simulink model "Project4_Simulink_individual"  (R2024b)
settings: Solver=ode4  StartTime=0.0  StopTime=3600  FixedStep=0.005  RelTol=1e-3
values from neighbouring files (symbols this model uses):
  ad = 2.5    [project4_code_final.m]
  b_capacity = 1500    [project4_code_final.m]
  c0 = 0.0041    [project4_code_final.m]
  c1 = 0.000066    (= 6.6e-05)    [project4_code_final.m]
  c_lambda = 50    [project4_code_final.m]
  calpha_front = 40000    [project4_code_final.m]
  calpha_rear = 40000    [project4_code_final.m]
  cd = 0.35    [project4_code_final.m]
  corner_factor = .95    (= 0.95)    [project4_code_final.m]
  eta_motor = 0.9    [project4_code_final.m]
  fyfrontmax = calpha_front * deg2rad(1)    [project4_code_final.m]
  fyrearmax = calpha_rear * deg2rad(1)    [project4_code_final.m]
  gratio = 2.5    [project4_code_final.m]
  i_gear_i = 0.005    [project4_code_final.m]
  inertia = 2000    [project4_code_final.m]
  ipt = 0.010    (= 0.01)    [project4_code_final.m]
  iw = 0.5 * 0.001* rw^2    (= 4.5e-05)    [project4_code_final.m]
  kd = 10000000    [project4_code_final.m]
  ki = 100    [project4_code_final.m]
  kp = 50000000    [project4_code_final.m]
  lambda_max = 0.1    [project4_code_final.m]
  lf = 1.0    (= 1)    [project4_code_final.m]
  lookahead_dist = 50    [project4_code_final.m]
  lookahead_dist_long = 100    [project4_code_final.m]
  lr = 1.5    [project4_code_final.m]
  mass = 1500    [project4_code_final.m]
  maxAlpha = 4 / 180 * pi    (= 0.0698131700798)    [project4_code_final.m]
  motor_torque_curve = [motor_rpm', motor_torque']    [project4_code_final.m]
  numSeries = 96    [project4_code_final.m]
  o_gear_i = 0.007    [project4_code_final.m]
  OCV = [0, 3.1,3.55,3.68,3.74,3.76,3.78,3.85,3.9,3.95,4.08,4.15]    [project4_code_final.m]
  omega0 = 0    [project4_code_final.m]
  psi0 = 0    [project4_code_final.m]
  r_internal = 0.1695    [project4_code_final.m]
  rho = 1.225    [project4_code_final.m]
  rw = 0.3    [project4_code_final.m]
  slope_angle_rad = atan(slope)    [project4_code_final.m]
  SOC = [0, 0.01,   .1,  .2,  .3,  .4,  .5,  .6, .7,  .8,  .9,   1]    [project4_code_final.m]
  soc_min = 0.1    [project4_code_final.m]
  T_lookahead = 0.3    [project4_code_final.m]
  tau_brakes = 50000    [project4_code_final.m]
  tire_mu = 1.0    (= 1)    [project4_code_final.m]
  v_batt = 350    [project4_code_final.m]
  vm = 1600    [project4_code_final.m]
  vx_threshold1 = 0.1    [project4_code_final.m]
  vxd = (max_motor_radps / gratio) * rw    [project4_code_final.m]
  vy0 = 0    [project4_code_final.m]
  wheelbase = lf + lr    (= 2.5)    [project4_code_final.m]
  x0 = 0    [project4_code_final.m]
  xpath = zeros(npts,1)    [project4_code_final.m]
  y0 = 0    [project4_code_final.m]
  ypath = zeros(npts,1)    [project4_code_final.m]
settings Model: Creator=btagl  LastModifiedBy=btagl

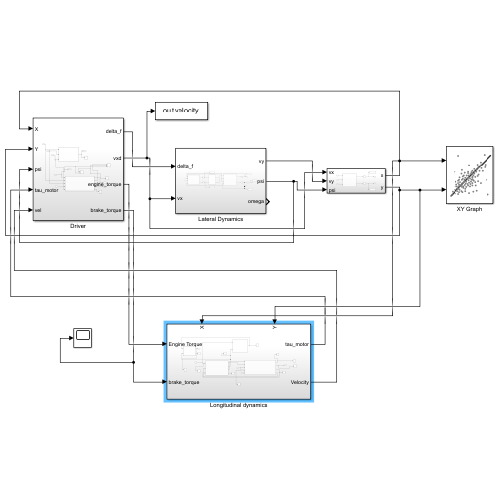
[thumbnail: Simulink's stored preview of the top-level diagram]
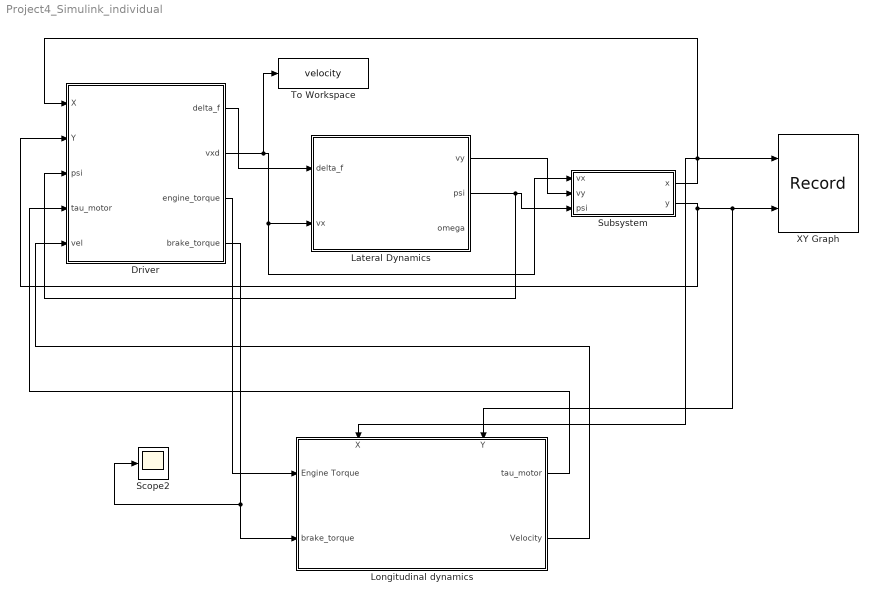
== system Project4_Simulink_individual ==
  Driver : Subsystem
  Lateral Dynamics : Subsystem
  Longitudinal dynamics : Subsystem
      settings: PortSchema="{\"entries\":[{\"content\":{\"sides\":[{\"content\":{\"connectorIds\":[\"In1\",\"In2\"]},\"type\":\"ConnectorPlacement.EquallySpacedRectSide\",\"uuid\":\"5c122f32-35de-43a9-a1a6-3743865a1a6c\"},{\"content\":{\"connectorIds\":[\"Out1\",\"Out2\"],\"side\":\"RIGHT\"},\"type\":\"ConnectorPlacement.EquallySpacedRectSide\",\"uuid\":\"4d44fb3e-15d5-4aaf-9487-b8861bfa0dad\"},{\"content\":{\"connectorIds\":[\"In3\",\"In4\"],\"side\":\"TOP\"},\"type\":\"ConnectorPlacement.EquallySpacedRectSide\",\"uuid\":\"e04a63df-9e81-4984-8ed3-9eee29f9a203\"}]},\"type\":\"ConnectorPlacement.EquallySpacedConnector\",\"uuid\":\"0a9d5385-60cd-4d4e-a9b3-28f03bd6bd4c\"}],\"packageUris\":[\"http://schema.mathworks.com/mf0/Connector/R2020b\"],\"version\":\"1.0\"}"
  Scope2 : Scope
  Subsystem : Subsystem
  To Workspace : ToWorkspace  VariableName=velocity  SaveFormat=Timeseries  SampleTime=-1
  XY Graph : Record  FileSettingsInternal="{\"entries\":[{\"content\":{\"excelSettings\":{\"content\":{},\"type\":\"Streamout.ExcelSettings\"}},\"type\":\"Streamout.FileSettingStorage\",\"uuid\":\"\"}],\"packageUris\":[\"http:\\/\\/schema.mathworks.com\\/mf0\\/streamout_blocks\\/R2020a\"],\"version\":\"1.0\"}"  Layout=[1 1]  SignalsInternal="{\"entries\":[{\"content\":{\"signals\":[{\"content\":{\"blockPath\":[],\"dimensions\":[1],\"domain\":\"\",\"lineColor\":\"#a2142f\",\"plots\":[ 1 ],\"port\":1,\"sid\":[\"\"],\"signalID\":1,\"signalName\":\"Subsystem:1\"},\"type\":\"RecordBlkView.Signal\",\"uuid\":\"\"},{\"content\":{\"blockPath\":[],\"dimensions\":[1],\"domain\":\"\",\"lineColor\":\"#139fff\",\"plots\":[ 1 ],\"port\":2,\"sid\":[\"\"],\"signalID\":2,\"signalName\":\"Subsystem:2\"},\"type\":\"RecordBlkView.Signal\",\"uuid\":\"\"}]},\"type\":\"RecordBlkView.InputSignals\",\"uuid\":\"\"}],\"packageUris\":[\"http:\\/\\/schema.mathworks.com\\/mf0\\/streamout_blocks\\/R2020a\"],\"version\":\"1.0\"}"  VisualizationBindings="{\"xyplotplugin\":{\"info\":[{\"series\":[{\"bindingParametersList\":[{\"parameter\":\"X-Axis\",\"signalID\":1,\"signalName\":\"Subsystem:1\"},{\"parameter\":\"Y-Axis\",\"signalID\":2,\"signalName\":\"Subsystem:2\"}],\"seriesID\":0}],\"subplotID\":1}]}}"  CompatibilityTag=XY
  wires:
  Subsystem/2(y) -> Driver/2(Y), XY Graph/2, Longitudinal dynamics/4(Y)
  Lateral Dynamics/2(psi) -> Driver/3(psi), Subsystem/3(psi)
  Lateral Dynamics/1(vy) -> Subsystem/2(vy)
  Driver/1(delta_f) -> Lateral Dynamics/1(delta_f)
  Driver/3(engine_torque) -> Longitudinal dynamics/1(Engine Torque)
  Driver/4(brake_torque) -> Scope2/1, Longitudinal dynamics/2(brake_torque)
  Longitudinal dynamics/1(tau_motor) -> Driver/4(tau_motor)
  Longitudinal dynamics/2(Velocity) -> Driver/5(vel)
  Driver/2(vxd) -> To Workspace/1, Subsystem/1(vx), Lateral Dynamics/2(vx)
  Subsystem/1(x) -> XY Graph/1, Longitudinal dynamics/3(X), Driver/1(X)

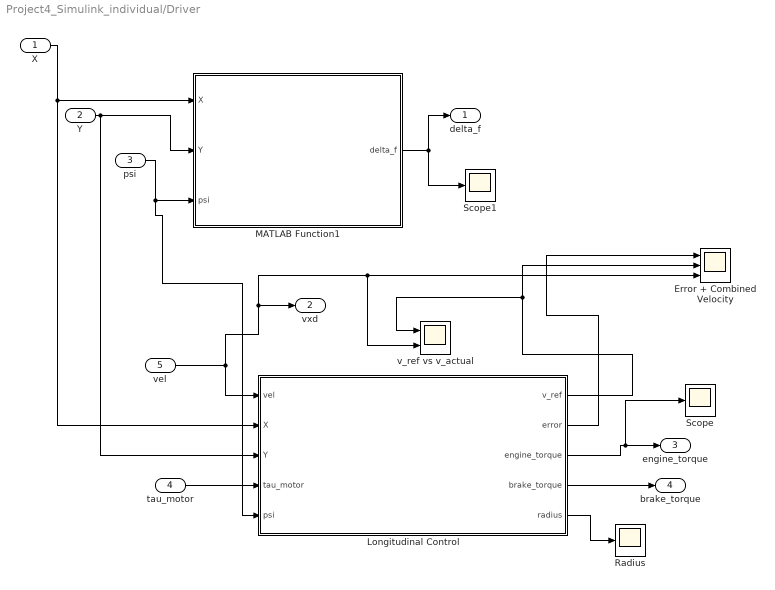
== system Project4_Simulink_individual/Driver ==
  X : Inport
  Y : Inport  Port=2
  psi : Inport  Port=3
  tau_motor : Inport  Port=4
  vel : Inport  Port=5
  Error + Combined Velocity : Scope  NumInputPorts=3
  Longitudinal Control : MATLAB Function  TreatAsAtomicUnit=on
  MATLAB Function1 : MATLAB Function  TreatAsAtomicUnit=on
  Radius : Scope
  Scope : Scope
  Scope1 : Scope
  v_ref vs v_actual : Scope  NumInputPorts=2
  delta_f : Outport
  vxd : Outport  Port=2
  engine_torque : Outport  Port=3
  brake_torque : Outport  Port=4
  wires:
  Y/1 -> Longitudinal Control/3(Y), MATLAB Function1/2(Y)
  X/1 -> Longitudinal Control/2(X), MATLAB Function1/1(X)
  MATLAB Function1/1(delta_f) -> delta_f/1, Scope1/1
  psi/1 -> Longitudinal Control/5(psi), MATLAB Function1/3(psi)
  tau_motor/1 -> Longitudinal Control/4(tau_motor)
  vel/1 -> Longitudinal Control/1(vel), vxd/1, v_ref vs v_actual/2, Error + Combined Velocity/3
  Longitudinal Control/1(v_ref) -> v_ref vs v_actual/1, Error + Combined Velocity/2
  Longitudinal Control/4(brake_torque) -> brake_torque/1
  Longitudinal Control/3(engine_torque) -> Scope/1, engine_torque/1
  Longitudinal Control/5(radius) -> Radius/1
  Longitudinal Control/2(error) -> Error + Combined Velocity/1

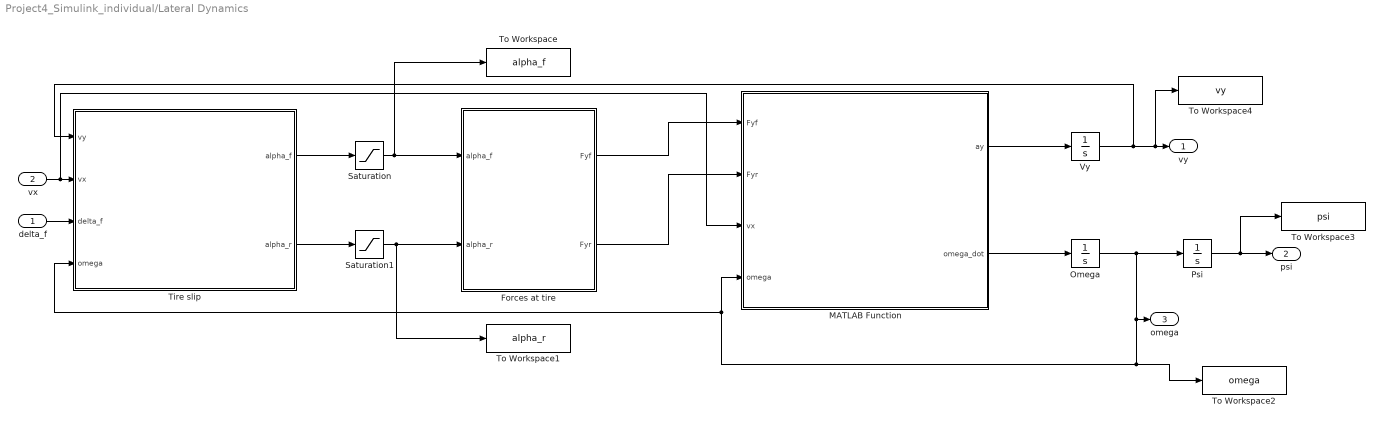
== system Project4_Simulink_individual/Lateral Dynamics ==
  delta_f : Inport
  vx : Inport  Port=2
  Forces at tire : MATLAB Function  TreatAsAtomicUnit=on
  MATLAB Function : MATLAB Function  TreatAsAtomicUnit=on
  Omega : Integrator  InitialCondition=omega0
  Psi : Integrator  InitialCondition=psi0
  Saturation : Saturate  UpperLimit=maxAlpha  LowerLimit=-maxAlpha
  Saturation1 : Saturate  UpperLimit=maxAlpha  LowerLimit=-maxAlpha
  Tire slip : MATLAB Function  TreatAsAtomicUnit=on
  To Workspace : ToWorkspace  VariableName=alpha_f  SaveFormat=Timeseries  SampleTime=-1
  To Workspace1 : ToWorkspace  VariableName=alpha_r  SaveFormat=Timeseries  SampleTime=-1
  To Workspace2 : ToWorkspace  VariableName=omega  SaveFormat=Timeseries  SampleTime=-1
  To Workspace3 : ToWorkspace  VariableName=psi  SaveFormat=Timeseries  SampleTime=-1
  To Workspace4 : ToWorkspace  VariableName=vy  SaveFormat=Timeseries  SampleTime=-1
  Vy : Integrator  InitialCondition=vy0
  vy : Outport
  psi : Outport  Port=2
  omega : Outport  Port=3
  wires:
  Tire slip/1(alpha_f) -> Saturation/1
  Tire slip/2(alpha_r) -> Saturation1/1
  delta_f/1 -> Tire slip/3(delta_f)
  vx/1 -> MATLAB Function/3(vx), Tire slip/2(vx)
  Saturation/1 -> To Workspace/1, Forces at tire/1(alpha_f)
  Saturation1/1 -> To Workspace1/1, Forces at tire/2(alpha_r)
  Forces at tire/1(Fyf) -> MATLAB Function/1(Fyf)
  Forces at tire/2(Fyr) -> MATLAB Function/2(Fyr)
  MATLAB Function/1(ay) -> Vy/1
  MATLAB Function/2(omega_dot) -> Omega/1
  Omega/1 -> Tire slip/4(omega), MATLAB Function/4(omega), To Workspace2/1, omega/1, Psi/1
  Psi/1 -> To Workspace3/1, psi/1
  Vy/1 -> Tire slip/1(vy), To Workspace4/1, vy/1

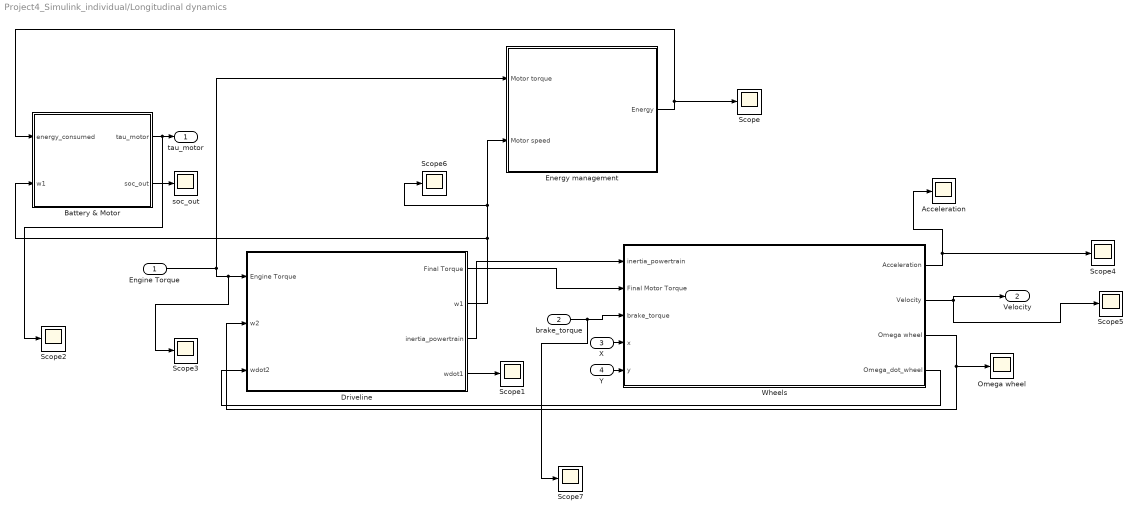
== system Project4_Simulink_individual/Longitudinal dynamics ==
  Engine Torque : Inport
  brake_torque : Inport  Port=2
  X : Inport  Port=3
  Y : Inport  Port=4
  Acceleration : Scope
  Battery & Motor : Subsystem
  Driveline : Subsystem
  Energy management : Subsystem
  Omega wheel : Scope
  Scope{,1..7} (8 alike) : Scope
  Wheels : Subsystem
  soc_out : Scope
  tau_motor : Outport
  Velocity : Outport  Port=2
  wires:
  Engine Torque/1 -> Energy management/1(Motor torque), Scope3/1, Driveline/1(Engine Torque)
  Driveline/1(Final Torque) -> Wheels/2(Final Motor Torque)
  Driveline/3(inertia_powertrain) -> Wheels/1(inertia_powertrain)
  brake_torque/1 -> Wheels/3(brake_torque), Scope7/1
  Wheels/1(Acceleration) -> Scope4/1, Acceleration/1
  Wheels/2(Velocity) -> Velocity/1, Scope5/1
  Wheels/4(Omega_dot_wheel) -> Driveline/3(wdot2)
  Wheels/3(Omega wheel) -> Driveline/2(w2), Omega wheel/1
  Driveline/2(w1) -> Battery & Motor/2(w1), Scope6/1, Energy management/2(Motor speed)
  Energy management/1(Energy) -> Scope/1, Battery & Motor/1(energy_consumed)
  Battery & Motor/2(soc_out) -> soc_out/1
  Battery & Motor/1(tau_motor) -> Scope2/1, tau_motor/1
  Driveline/4(wdot1) -> Scope1/1
  X/1 -> Wheels/4(x)
  Y/1 -> Wheels/5(y)

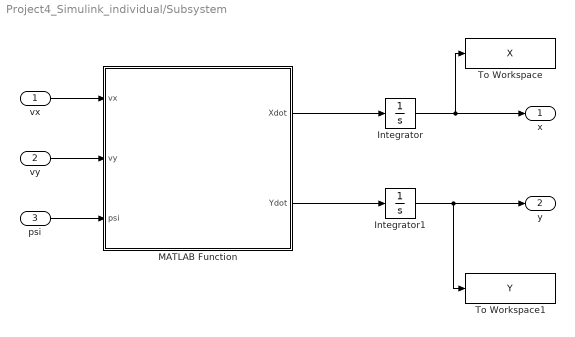
== system Project4_Simulink_individual/Subsystem ==
  vx : Inport
  vy : Inport  Port=2
  psi : Inport  Port=3
  Integrator : Integrator  InitialCondition=x0
  Integrator1 : Integrator  InitialCondition=y0
  MATLAB Function : MATLAB Function  TreatAsAtomicUnit=on
  To Workspace : ToWorkspace  VariableName=X  SaveFormat=Timeseries  SampleTime=-1
  To Workspace1 : ToWorkspace  VariableName=Y  SaveFormat=Timeseries  SampleTime=-1
  x : Outport
  y : Outport  Port=2
  wires:
  vx/1 -> MATLAB Function/1(vx)
  vy/1 -> MATLAB Function/2(vy)
  psi/1 -> MATLAB Function/3(psi)
  MATLAB Function/1(Xdot) -> Integrator/1
  MATLAB Function/2(Ydot) -> Integrator1/1
  Integrator/1 -> To Workspace/1, x/1
  Integrator1/1 -> To Workspace1/1, y/1

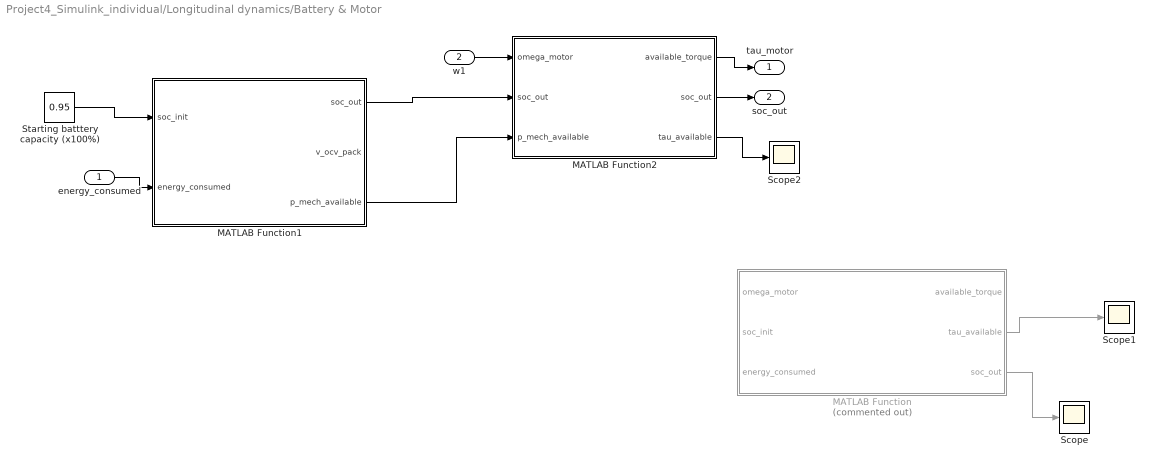
== system Project4_Simulink_individual/Longitudinal dynamics/Battery & Motor ==
  energy_consumed : Inport
  w1 : Inport  Port=2
  MATLAB Function : MATLAB Function  Commented=on  TreatAsAtomicUnit=on
  MATLAB Function1 : MATLAB Function  TreatAsAtomicUnit=on
  MATLAB Function2 : MATLAB Function  TreatAsAtomicUnit=on
  Scope : Scope
  Scope1 : Scope
  Scope2 : Scope
  Starting batttery capacity (x100%) : Constant  Value=0.95
  tau_motor : Outport
  soc_out : Outport  Port=2
  wires:
  MATLAB Function/3(soc_out) -> Scope/1
  MATLAB Function/2(tau_available) -> Scope1/1
  energy_consumed/1 -> MATLAB Function1/2(energy_consumed)
  Starting batttery capacity (x100%)/1 -> MATLAB Function1/1(soc_init)
  MATLAB Function1/3(p_mech_available) -> MATLAB Function2/3(p_mech_available)
  MATLAB Function1/1(soc_out) -> MATLAB Function2/2("soc_out ")
  w1/1 -> MATLAB Function2/1(omega_motor)
  MATLAB Function2/1(available_torque) -> tau_motor/1
  MATLAB Function2/2(soc_out) -> soc_out/1
  MATLAB Function2/3(tau_available) -> Scope2/1

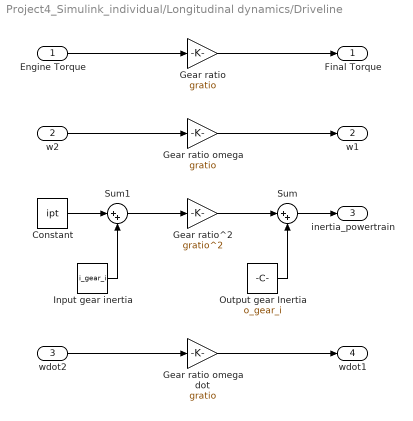
== system Project4_Simulink_individual/Longitudinal dynamics/Driveline ==
  Engine Torque : Inport
  w2 : Inport  Port=2
  wdot2 : Inport  Port=3
  Constant : Constant  Value=ipt
  Gear ratio : Gain  Gain=gratio
  Gear ratio omega : Gain  Gain=gratio
  Gear ratio omega dot : Gain  Gain=gratio
  Gear ratio^2 : Gain  Gain=gratio^2
  Input gear inertia : Constant  Value=i_gear_i
  Output gear Inertia : Constant  Value=o_gear_i
  Sum : Sum  Inputs=|++
  Sum1 : Sum  Inputs=|++
  Final Torque : Outport
  w1 : Outport  Port=2
  inertia_powertrain : Outport  Port=3
  wdot1 : Outport  Port=4
  wires:
  Engine Torque/1 -> Gear ratio/1
  Gear ratio/1 -> Final Torque/1
  Gear ratio omega/1 -> w1/1
  w2/1 -> Gear ratio omega/1
  Input gear inertia/1 -> Sum1/2
  Constant/1 -> Sum1/1
  Sum1/1 -> Gear ratio^2/1
  Output gear Inertia/1 -> Sum/2
  Gear ratio^2/1 -> Sum/1
  Sum/1 -> inertia_powertrain/1
  Gear ratio omega dot/1 -> wdot1/1
  wdot2/1 -> Gear ratio omega dot/1

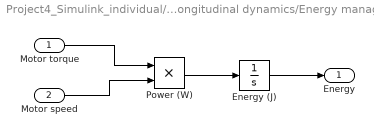
== system Project4_Simulink_individual/Longitudinal dynamics/Energy management ==
  Motor torque : Inport
  Motor speed : Inport  Port=2
  Energy (J) : Integrator
  Power (W) : Product
  Energy : Outport
  wires:
  Motor torque/1 -> Power (W)/1
  Motor speed/1 -> Power (W)/2
  Power (W)/1 -> Energy (J)/1
  Energy (J)/1 -> Energy/1

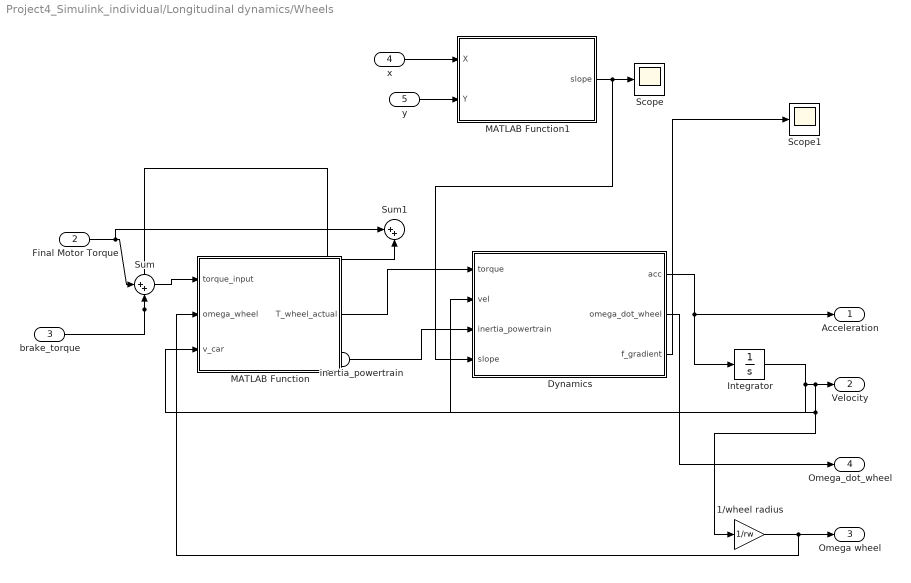
== system Project4_Simulink_individual/Longitudinal dynamics/Wheels ==
  inertia_powertrain : Inport
  Final Motor Torque : Inport  Port=2
  brake_torque : Inport  Port=3
  x : Inport  Port=4
  y : Inport  Port=5
  1/wheel radius : Gain  Gain=1/rw
  Dynamics : MATLAB Function  TreatAsAtomicUnit=on
  Integrator : Integrator
  MATLAB Function : MATLAB Function  TreatAsAtomicUnit=on
  MATLAB Function1 : MATLAB Function  TreatAsAtomicUnit=on
  Scope : Scope
  Scope1 : Scope
  Sum : Sum  Inputs=|++
  Sum1 : Sum  Inputs=|++
  Acceleration : Outport
  Velocity : Outport  Port=2
  Omega wheel : Outport  Port=3
  Omega_dot_wheel : Outport  Port=4
  wires:
  Dynamics/1(acc) -> Integrator/1, Acceleration/1
  Integrator/1 -> Dynamics/2(vel), MATLAB Function/3(v_car), 1/wheel radius/1, Velocity/1
  inertia_powertrain/1 -> Dynamics/3(inertia_powertrain)
  Dynamics/2(omega_dot_wheel) -> Omega_dot_wheel/1
  1/wheel radius/1 -> MATLAB Function/2(omega_wheel), Omega wheel/1
  Final Motor Torque/1 -> Sum1/1, Sum/1
  brake_torque/1 -> Sum/2, Sum1/2
  Sum/1 -> MATLAB Function/1(torque_input)
  MATLAB Function/1(T_wheel_actual) -> Dynamics/1(torque)
  MATLAB Function1/1(slope) -> Dynamics/4(slope), Scope/1
  x/1 -> MATLAB Function1/1(X)
  y/1 -> MATLAB Function1/2(Y)
  Dynamics/3(f_gradient) -> Scope1/1

== matlab function Project4_Simulink_individual/Driver/Longitudinal Control ==
  settings: updateMethod=DISCRETE
  data: vel input; v_ref output; X input; Y input; xpath parameter; ypath parameter; mass parameter; fyfrontmax parameter; fyrearmax parameter; kp parameter; ki parameter; kd parameter; tau_brakes parameter; tau_motor input; error output; engine_torque output; brake_torque output; lookahead_dist_long parameter; vxd parameter; corner_factor parameter; wheelbase parameter; T_lookahead parameter; radius output; psi input
function [v_ref, error, engine_torque, brake_torque, radius] = driver_model_predictive_steering(...
    vel, X, Y, xpath, ypath, ...
    mass, fyfrontmax, fyrearmax, ...
    kp, ki, kd, tau_brakes, tau_motor, ...
    lookahead_dist_long, vxd, corner_factor, wheelbase, T_lookahead, psi)

    % Speed-based minimum friction braking percentage
    v_mph = vel * 2.23694;  % Convert m/s to mph
    
    if v_mph <= 5
        friction_pct = 1.0;
    elseif v_mph < 25
        friction_pct = 1.0 - 0.95 * (v_mph - 5) / 20;  
    else
        friction_pct = 0.05;
    end
    
    regen_pct = 1.0 - friction_pct;
    tau_regen_max = tau_motor * regen_pct;
        
    % Persistent variables for PID
    persistent integral_error prev_error;
    if isempty(integral_error)
        integral_error = 0;
        prev_error = 0;
    end

    % -------- Predictive Pose --------
    X_pred = X + vel * T_lookahead * cos(psi);
    Y_pred = Y + vel * T_lookahead * sin(psi);
    psi_pred = psi;

    % -------- Pure Pursuit to Predict Steering --------
    delta_f_pred = compute_delta_f(X_pred, Y_pred, psi_pred, wheelbase, lookahead_dist_long, xpath, ypath);

    % -------- Radius from Predicted delta_f --------
    if abs(tan(delta_f_pred)) > 1e-4
        radius = wheelbase / tan(abs(delta_f_pred));
        kappa = 1 / radius;
    else
        radius = Inf;
        kappa = 0;
    end

    % -------- Reference Velocity --------
    Fy_total_max = fyfrontmax + fyrearmax;
    ay_max = Fy_total_max / mass;

    if kappa > 1e-6
        v_ref = sqrt(ay_max / kappa) * corner_factor;
    else
        v_ref = vxd;
    end

    % -------- PID Control --------
    error = v_ref - vel;
    integral_error = integral_error + error;
    derivative_error = error - prev_error;
    prev_error = error;

    alpha_driver = kp * error + ki * integral_error + kd * derivative_error;
    alpha_driver = max(-1, min(1, alpha_driver));

    % -------- Torque Output --------
    if alpha_driver >= 0
        engine_torque = alpha_driver * tau_motor;
        brake_torque = 0;
    else
        brake_total = -alpha_driver * tau_brakes;
        regen = min(brake_total, tau_regen_max);
        engine_torque = -regen;
        brake_torque = -(brake_total - regen);
    end
end

% ---------------- Nested Pure Pursuit Function ----------------
function delta_f = compute_delta_f(X, Y, psi, wheelbase, lookahead_dist, xpath, ypath)
    delta_f = 0;
    xt = X;
    yt = Y;
    min_valid_dist = Inf;

    for i = 1:length(xpath)
        dx = xpath(i) - X;
        dy = ypath(i) - Y;

        % Transform to vehicle coordinates
        x_local = cos(psi) * dx + sin(psi) * dy;
        y_local = -sin(psi) * dx + cos(psi) * dy;

        dist = sqrt(dx^2 + dy^2);

        if (x_local > 0) && (dist >= lookahead_dist) && (dist < min_valid_dist)
            xt = xpath(i);
            yt = ypath(i);
            min_valid_dist = dist;
        end
    end

    if min_valid_dist < Inf
        dx = xt - X;
        dy = yt - Y;

        x_local = cos(psi) * dx + sin(psi) * dy;
        y_local = -sin(psi) * dx + cos(psi) * dy;

        curvature = (2 * y_local) / (lookahead_dist^2);
        delta_f = atan(wheelbase * curvature);
    end
end

== matlab function Project4_Simulink_individual/Longitudinal dynamics/Wheels/Dynamics ==
  data: acc output; torque input; iw parameter; rw parameter; vm parameter; cd parameter; vel input; ad parameter; rho parameter; inertia_powertrain input; omega_dot_wheel output; c0 parameter; c1 parameter; f_gradient output; slope input
function [acc, omega_dot_wheel,f_gradient] = fcn(torque, iw, rw, vm, cd,vel,ad,rho, inertia_powertrain,c0, c1,slope)

fdrag=0.5*(rho*ad*cd*vel^2);
frr=c0+c1*vel;
meq=((inertia_powertrain+iw)/rw^2)+vm;
f_gradient=vm*9.81*sin(slope);
fx=(torque/rw)-fdrag-frr-f_gradient;
acc=(fx/meq);
omega_dot_wheel=acc/rw; %rad/s^2 angular acceleration

== matlab function Project4_Simulink_individual/Longitudinal dynamics/Battery & Motor/MATLAB Function ==
  data: omega_motor input; v_batt parameter; r_internal parameter; eta_motor parameter; soc_min parameter; soc_init input; motor_torque_curve parameter; energy_consumed input; b_capacity parameter; available_torque output; tau_available output; soc_out output
function [available_torque, tau_available, soc_out] = compute_available_torque(...
    omega_motor, v_batt, r_internal, eta_motor, soc_min, soc_init, ...
    motor_torque_curve, energy_consumed, b_capacity)

    % Convert omega (rad/s) to RPM
    rpm_motor = omega_motor * 60 / (2 * pi);

    % Lookup motor torque limit at current RPM
    tau_motor_limit = interp1(motor_torque_curve(:,1), motor_torque_curve(:,2), ...
                              rpm_motor, 'linear', 'extrap');

    % Compute SOC based on energy used so far
    soc_out = soc_init - (energy_consumed / (3600 * v_batt * b_capacity));
    soc_out = max(soc_min, soc_out);  % prevent dropping below min

    % Default torque values
    available_torque = 0;
    tau_available = 0;

    % Case 1: SOC too low
    if soc_out <= soc_min
        return;

    % Case 2: Motor is stalled
    elseif omega_motor < 1e-3
        available_torque = tau_motor_limit;
        tau_available = available_torque;

    % Case 3: Power-limited torque
    else
        p_max_batt = (v_batt^2) / (4 * r_internal);
        p_mech_available = p_max_batt * eta_motor;
        tau_available_batt = p_mech_available / omega_motor;

        % Final torque = limited by both motor and battery
        available_torque = min(tau_available_batt, tau_motor_limit);
        tau_available = tau_available_batt;
    end
end

== matlab function Project4_Simulink_individual/Longitudinal dynamics/Battery & Motor/MATLAB Function1 ==
  data: soc_out output; v_ocv_pack output; soc_init input; energy_consumed input; soc_min parameter; SOC parameter; OCV parameter; numSeries parameter; r_internal parameter; eta_motor parameter; p_mech_available output; b_capacity parameter
function [soc_out, v_ocv_pack, p_mech_available] = compute_battery_state(...
    soc_init, energy_consumed, soc_min, SOC, OCV, ...
    numSeries, r_internal, eta_motor, b_capacity)


    soc_out = soc_init - (energy_consumed / (3600 * b_capacity * mean(OCV) * numSeries));
    soc_out = max(soc_min, soc_out); % Clamp SOC at minimum

    v_cell = interp1(SOC, OCV, soc_out, 'linear', 'extrap');

    v_ocv_pack = v_cell * numSeries;

    r_total = r_internal; 

    % Maximum power transfer theorem: max power = (V_ocv)^2 / (4 * R)
    p_max_batt = (v_ocv_pack^2) / (4 * r_total);

    p_mech_available = p_max_batt * eta_motor;

end

== matlab function Project4_Simulink_individual/Longitudinal dynamics/Battery & Motor/MATLAB Function2 ==
  data: omega_motor input; available_torque output; soc_out output; soc_out input; p_mech_available input; tau_available output; motor_torque_curve parameter; soc_min parameter
function [available_torque, soc_out, tau_available] = compute_motor_torque(...
    omega_motor, soc_out, p_mech_available, motor_torque_curve, soc_min)

    % Convert omega (rad/s) to RPM
    rpm_motor = omega_motor * 60 / (2 * pi);

    % Lookup motor torque limit at current RPM
    tau_motor_limit = interp1(motor_torque_curve(:,1), motor_torque_curve(:,2), ...
                              rpm_motor, 'linear', 'extrap');

    % Default torque values
    available_torque = 0;
    tau_available = 0;

    % Case 1: SOC too low
    if soc_out <= soc_min
        return;

    % Case 2: Motor is stalled
    elseif omega_motor < 1e-3
        available_torque = tau_motor_limit;
        tau_available = available_torque;

    % Case 3: Power-limited torque
    else
        tau_available_batt = p_mech_available / omega_motor;
        available_torque = min(tau_available_batt, tau_motor_limit);
        tau_available = tau_available_batt;
    end
end

== matlab function Project4_Simulink_individual/Longitudinal dynamics/Wheels/MATLAB Function1 ==
  data: slope output; xpath parameter; ypath parameter; slope_angle_rad parameter; X input; Y input
function slope = get_slope_angle(xpath, ypath, slope_angle_rad, X, Y)
% Find closest track point
min_dist = Inf;
index = 1;
for i = 1:length(xpath)
    dx = xpath(i) - X;
    dy = ypath(i) - Y;
    dist = dx^2 + dy^2;

    if dist < min_dist
        min_dist = dist;
        index = i;
    end
end

slope = slope_angle_rad(index);  % Output in radians

== matlab function Project4_Simulink_individual/Lateral Dynamics/Tire slip ==
  data: vy input; alpha_f output; vx input; delta_f input; omega input; alpha_r output; lr parameter; lf parameter; vx_threshold1 parameter
function [alpha_f, alpha_r] = fcn(vy,  vx, delta_f, omega, lr, lf, vx_threshold1)


if abs(vx)> vx_threshold1
      alpha_f = delta_f - (vy + omega * lf) / vx;
      alpha_r = - (vy - omega * lr) / vx;
else
      alpha_f = 0;
      alpha_r = 0;
end



end

== matlab function Project4_Simulink_individual/Longitudinal dynamics/Wheels/MATLAB Function ==
  data: torque_input input; omega_wheel input; T_wheel_actual output; v_car input; mass parameter; rw parameter; c_lambda parameter; lambda_max parameter; tire_mu parameter
function T_wheel_actual = tire_slip_model(torque_input, omega_wheel, v_car, mass, rw, c_lambda, lambda_max, tire_mu)

g = 9.81; % [m/s²] gravity

F_desired = torque_input / rw;

% Calculate wheel linear speed
v_wheel = omega_wheel * rw;

% Calculate slip (protect against divide by zero)
if abs(v_car) < 0.5
    lambda = 0;
else
    lambda = (v_wheel - v_car) / v_car;
end

% Tire force limit ONLY if slip exceeds maximum
if abs(lambda) < lambda_max
    % Slip is under control → no need to clip the force
    F_actual = F_desired;
else
    % Slip exceeds max → limit force to available friction
    F_tire_max = tire_mu * mass * g;
    if abs(F_desired) <= F_tire_max
        F_actual = F_desired;
    else
        F_actual = sign(F_desired) * F_tire_max;
    end
end

% Output torque
T_wheel_actual = F_actual * rw;

end

== matlab function Project4_Simulink_individual/Lateral Dynamics/Forces at tire ==
  data: alpha_f input; Fyf output; alpha_r input; Fyr output; calpha_front parameter; calpha_rear parameter; fyfrontmax parameter; fyrearmax parameter
function [Fyf, Fyr] = fcn(alpha_f, alpha_r, calpha_front, calpha_rear, fyfrontmax, fyrearmax)

Fyf = min(fyfrontmax,calpha_front * alpha_f);
Fyr = min(fyrearmax, calpha_rear * alpha_r);
end

== matlab function Project4_Simulink_individual/Lateral Dynamics/MATLAB Function ==
  data: Fyf input; ay output; Fyr input; vx input; omega input; omega_dot output; lf parameter; lr parameter; inertia parameter; mass parameter
function [ay, omega_dot] = fcn(Fyf, Fyr, vx, omega, lf, lr, inertia, mass)

Fy = Fyf + Fyr;
ay = Fy / mass - omega * vx;
        
M  = Fyf * lf - Fyr * lr;        
omega_dot = M / inertia;        

end

== matlab function Project4_Simulink_individual/Subsystem/MATLAB Function ==
  data: vx input; Xdot output; vy input; psi input; Ydot output
function [Xdot, Ydot] = fcn(vx, vy, psi)
    temp = TF(psi) * [vx;vy]; 
    Xdot = temp(1);
    Ydot = temp(2);
  
end

function y = TF(psi)
    y = [cos(psi), -sin(psi); sin(psi), cos(psi)];
end

== matlab function Project4_Simulink_individual/Driver/MATLAB Function1 ==
  data: X input; Y input; psi input; wheelbase parameter; lookahead_dist parameter; delta_f output; xpath parameter; ypath parameter
function delta_f = latControl_pure_pursuit(X, Y, psi, wheelbase, lookahead_dist, xpath, ypath)
    % Default steering angle
    delta_f = 0;

    % Default values for target
    xt = X;
    yt = Y;

    % Set large initial distance
    min_valid_dist = Inf;

    for i = 1:length(xpath)
        dx = xpath(i) - X;
        dy = ypath(i) - Y;

        % Transform to vehicle coordinates (ψ = + counter-clockwise)
        x_local = cos(psi) * dx + sin(psi) * dy;
        y_local = -sin(psi) * dx + cos(psi) * dy;

        dist = sqrt(dx^2 + dy^2);

        % Find closest valid point ahead of vehicle
        if (x_local > 0) && (dist >= lookahead_dist) && (dist < min_valid_dist)
            xt = xpath(i);
            yt = ypath(i);
            min_valid_dist = dist;
        end
    end

    % If target updated, compute steering
    if min_valid_dist < Inf
        dx = xt - X;
        dy = yt - Y;

        % Transform to vehicle frame again for y_local
        x_local = cos(psi) * dx + sin(psi) * dy;
        y_local = -sin(psi) * dx + cos(psi) * dy;

        curvature = (2 * y_local) / (lookahead_dist^2);
        delta_f = atan(wheelbase * curvature);
    end
end
